simulink model "ct"  (R2020a)
settings: Solver=VariableStepAuto  StartTime=0.0  StopTime=10.0  RelTol=1e-3
settings Model: Creator=lphoo  LastModifiedBy=lphoo

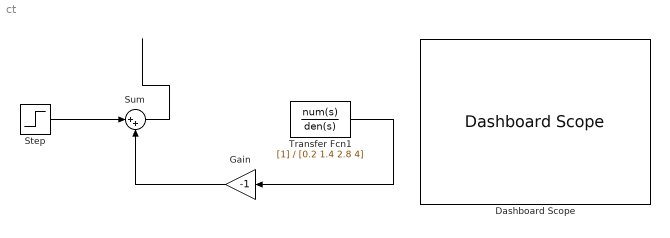
== system ct ==
  Dashboard Scope : DashboardScope  Ymin=0  Ymax=1.2
  Gain : Gain  Gain=-1
  Step : Step  SampleTime=0.01
  Sum : Sum  Inputs=|++
  Transfer Fcn1 : TransferFcn  Denominator=[0.2 1.4 2.8 4]  ContinuousStateAttributes=Plant
  wires:
  Gain/1 -> Sum/2
  Step/1 -> Sum/1
  Transfer Fcn1/1 -> Gain/1
  Sum/1 -> ?
